simulink model "robot5"  (R2016b)
settings: Solver=ode3  StartTime=0.0  StopTime=inf  RelTol=1e-3  EnableMultiTasking=on
libraries: vexarmcortexlib x20
settings Model: ExtModeTrigDuration=25  Creator=Betrh  LastModifiedBy=Otsubo
settings DataIOCC: LimitDataPoints=on  SignalLoggingSaveFormat=ModelDataLogs
settings OptimizationCC: ExpressionDepthLimit=2147483647  LifeSpan=Inf  MaxStackSize=64
settings DebuggingCC: UnderspecifiedInitializationDetection=Classic  MergeDetectMultiDrivingBlocksExec=none  InheritedTsInSrcMsg=none  FcnCallInpInsideContextMsg=warning  UnconnectedInputMsg=none  UnconnectedOutputMsg=none  StateNameClashWarn=warning  SFUnexpectedBacktrackingDiag=warning  SFNoUnconditionalDefaultTransitionDiag=warning  SFExecutionAtInitializationDiag=none
settings HardwareCC: ProdBitPerPointer=32  ProdBitPerSizeT=32  ProdBitPerPtrDiffT=32  ProdLargestAtomicInteger=Long  ProdLargestAtomicFloat=Double  ProdIntDivRoundTo=Undefined  ProdWordSize=32  ProdHWDeviceType=ARM Compatible->ARM Cortex
settings ModelReferenceCC: PropagateSignalLabelsOutOfModel=off
settings RTWCC: SystemTargetFile=ert.tlc  HardwareBoard=ARM Cortex-based VEX Microcontroller  TemplateMakefile=ert_default_tmf  Description=Embedded Coder  Toolchain=GNU Tools for VEX ARM Cortex
settings CodeAppCC: IgnoreCustomStorageClasses=off  CustomSymbolStrType=$N$R$M  InternalIdentifier=Classic
settings ERTTargetCC: CodeReplacementLibrary=GCC ARM Cortex-M3  ConvertIfToSwitch=off  SuppressUnreachableDefaultCases=off

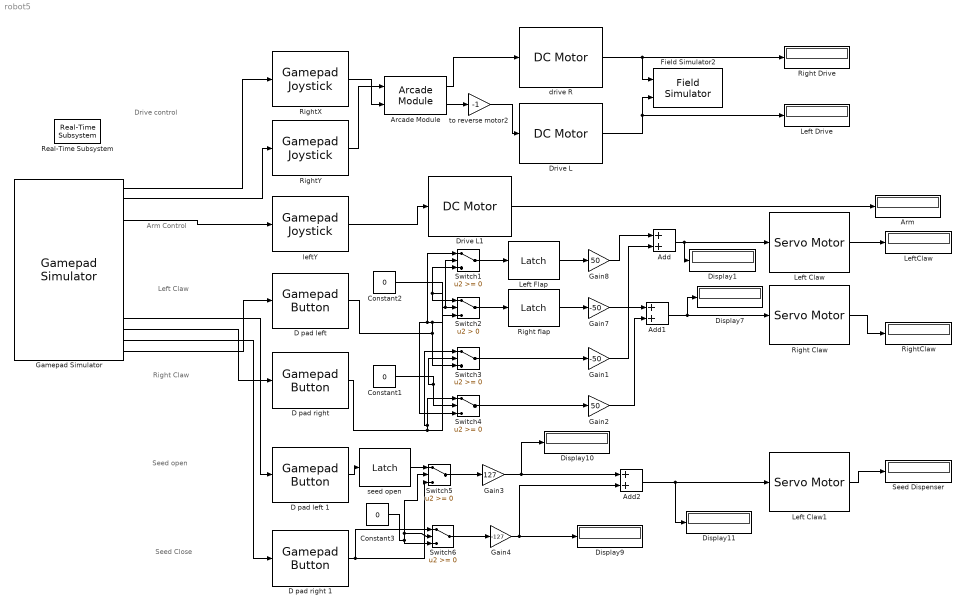
== system robot5 ==
  note: Left Claw
  note: Arm Control
  note: Drive control
  note: Seed Close
  note: Right Claw
  note: Seed open
  Add : Sum
  Add1 : Sum
  Add2 : Sum
  Arcade Module : vexarmcortexlib/Utilities/Arcade Module
  Arm : Display
  Constant1 : Constant  Value=0
  Constant2 : Constant  Value=0
  Constant3 : Constant  Value=0
  "D pad left " : vexarmcortexlib/Gamepad Button  joystick=1  chan=7  button56=Up  button78=Left  SimulationIn=on  sample_time=-1
  D pad left 1 : vexarmcortexlib/Gamepad Button  joystick=1  chan=7  button56=Up  button78=Up  SimulationIn=on  sample_time=-1
  "D pad right " : vexarmcortexlib/Gamepad Button  joystick=1  chan=7  button56=Up  button78=Right  SimulationIn=on  sample_time=-1
  D pad right 1 : vexarmcortexlib/Gamepad Button  joystick=1  chan=7  button56=Up  button78=Down  SimulationIn=on  sample_time=-1
  Display{1,7,9..11} (5 alike) : Display
  Drive L : vexarmcortexlib/DC Motor  motor=2  scaleFactor=1/13.5  SimulationOut=on
  Drive L1 : vexarmcortexlib/DC Motor  motor=4  scaleFactor=1/13.5  SimulationOut=on
  Field Simulator2 : vexarmcortexlib/Utilities/Field Simulator  radius=2.5  space=10  range=200
  Gain1 : Gain  Gain=-50
  Gain2 : Gain  Gain=50
  Gain3 : Gain  Gain=127
  Gain4 : Gain  Gain=-127
  Gain7 : Gain  Gain=-50
  Gain8 : Gain  Gain=50
  Gamepad Simulator : vexarmcortexlib/Utilities/Gamepad Simulator  WhichPad=Logitech Gamepad  JoyId=1
  Left Claw : vexarmcortexlib/Servo Motor  motor=5  scaleFactor=60/127  SimulationOut=on
  Left Claw1 : vexarmcortexlib/Servo Motor  motor=5  scaleFactor=60/127  SimulationOut=on
  Left Drive : Display
  "Left Flap " : vexarmcortexlib/Utilities/Latch  output0=off
  LeftClaw : Display
  Real-Time Subsystem : vexarmcortexlib/Utilities/Real-Time Subsystem  x=1
  Right Claw : vexarmcortexlib/Servo Motor  motor=6  scaleFactor=60/127  SimulationOut=on
  Right Drive : Display
  "Right flap " : vexarmcortexlib/Utilities/Latch  output0=off
  RightClaw : Display
  "RightX " : vexarmcortexlib/Gamepad Joystick  joystick=1  chan=1  SimulationIn=on  sample_time=-1
  RightY : vexarmcortexlib/Gamepad Joystick  joystick=1  chan=2  SimulationIn=on  sample_time=-1
  Seed Dispenser : Display
  Switch{1,3..6} (5 alike) : Switch
  Switch2 : Switch  Criteria=u2 > Threshold
  drive R : vexarmcortexlib/DC Motor  motor=1  scaleFactor=1/13.5  SimulationOut=on
  leftY : vexarmcortexlib/Gamepad Joystick  joystick=1  chan=4  SimulationIn=on  sample_time=-1
  seed open : vexarmcortexlib/Utilities/Latch  output0=off
  to reverse motor2 : Gain  Gain=-1
  wires:
  Gamepad Simulator/16 -> "D pad left "/1
  Gamepad Simulator/14 -> "D pad right "/1
  Arcade Module/2 -> to reverse motor2/1
  drive R/1 -> Right Drive/1, Field Simulator2/1
  Drive L1/1 -> Arm/1
  Drive L/1 -> Field Simulator2/2, Left Drive/1
  Gamepad Simulator/4 -> leftY/1
  Left Claw/1 -> LeftClaw/1
  Right Claw/1 -> RightClaw/1
  "RightX "/1 -> Arcade Module/2
  RightY/1 -> Arcade Module/1
  Switch1/1 -> "Left Flap "/1
  Switch2/1 -> "Right flap "/1
  "Left Flap "/1 -> Gain8/1
  Switch3/1 -> Gain1/1
  "D pad left "/1 -> Switch4/3, Switch1/1, Switch2/3, Switch3/3
  Constant2/1 -> Switch1/2, Switch2/2
  "D pad right "/1 -> Switch1/3, Switch2/1, Switch3/1, Switch4/1
  "Right flap "/1 -> Gain7/1
  Switch4/1 -> Gain2/1
  Constant1/1 -> Switch4/2, Switch3/2
  Gain1/1 -> Add/2
  Gain2/1 -> Add1/2
  Gain8/1 -> Add/1
  Gain7/1 -> Add1/1
  Add1/1 -> Display7/1, Right Claw/1
  Add/1 -> Display1/1, Left Claw/1
  Gamepad Simulator/1 -> "RightX "/1
  Gamepad Simulator/2 -> RightY/1
  Arcade Module/1 -> drive R/1
  to reverse motor2/1 -> Drive L/1
  Gamepad Simulator/13 -> D pad left 1/1
  Gamepad Simulator/15 -> D pad right 1/1
  D pad left 1/1 -> seed open/1
  Constant3/1 -> Switch5/2, Switch6/2, Switch6/3
  seed open/1 -> Switch5/1
  Switch5/1 -> Gain3/1
  D pad right 1/1 -> Switch5/3, Switch6/1
  Gain3/1 -> Add2/1, Display10/1
  Switch6/1 -> Gain4/1
  Gain4/1 -> Add2/2, Display9/1
  Add2/1 -> Display11/1, Left Claw1/1
  Left Claw1/1 -> Seed Dispenser/1
  leftY/1 -> Drive L1/1
